simulink model "quadcopter_wind_adaptive_AW"  (R2017b)
settings: Solver=ode45  StartTime=0.0  StopTime=100  FixedStep=0.001  RelTol=1e-3  EnableMultiTasking=on
values from neighbouring files (symbols this model uses):
  aw = 1    [control_params.m]
  C = 1    [control_params.m]
  f_phi = 0.01    [control_params.m]
  f_psi = 0.01    [control_params.m]
  f_theta = 0.01    [control_params.m]
  f_x = 0.01    [control_params.m]
  f_y = 0.01    [control_params.m]
  f_z = 0.01    [control_params.m]
  g = 9.8    [control_params.m]
  J_1 = 0.02    [control_params.m]
  J_2 = 0.02    [control_params.m]
  J_3 = 0.01    [control_params.m]
  l = 0.2    [control_params.m]
  lim_phi = 0.1    [control_params.m]
  lim_psi = 0.1    [control_params.m]
  lim_theta = 0.1    [control_params.m]
  lim_x = 0.1    [control_params.m]
  lim_y = 0.1    [control_params.m]
  lim_z = 6    [control_params.m]
  m = 0.5    [control_params.m]
  phi_desired = 1    [control_params.m]
  x_desired = 1    [control_params.m]
  y_desired = 1    [control_params.m]
  z_desired = 1    [control_params.m]
settings Model: Creator=Oleg Borisov  LastModifiedBy=broth
settings DataIOCC: LimitDataPoints=on  SaveFormat=Array  SignalLoggingSaveFormat=ModelDataLogs
settings OptimizationCC: ExpressionDepthLimit=2147483647  LifeSpan=inf
settings DebuggingCC: UnderspecifiedInitializationDetection=Classic  MergeDetectMultiDrivingBlocksExec=none  SolverPrmCheckMsg=warning  FcnCallInpInsideContextMsg=warning  StateNameClashWarn=warning  SFUnexpectedBacktrackingDiag=warning  SFNoUnconditionalDefaultTransitionDiag=warning  SFExecutionAtInitializationDiag=none
settings HardwareCC: ProdBitPerPointer=32  ProdBitPerSizeT=32  ProdBitPerPtrDiffT=32  ProdLargestAtomicFloat=None  ProdIntDivRoundTo=Undefined  ProdEndianess=Unspecified  ProdWordSize=32  ProdHWDeviceType=32-bit Generic
settings ModelReferenceCC: PropagateSignalLabelsOutOfModel=off
settings CodeAppCC: StateflowObjectComments=on
settings GRTTargetCC: TargetLangStandard=C89/C90 (ANSI)  GeneratePreprocessorConditionals=Disable all  CombineOutputUpdateFcns=off  GRTInterface=on
settings ConfigComp: CovMetricSettings=dw  CovHtmlReporting=on  CovSaveCumulativeToWorkspaceVar=on  CovSaveSingleToWorkspaceVar=on  CovExternalEMLEnable=off  CovSFcnEnable=off

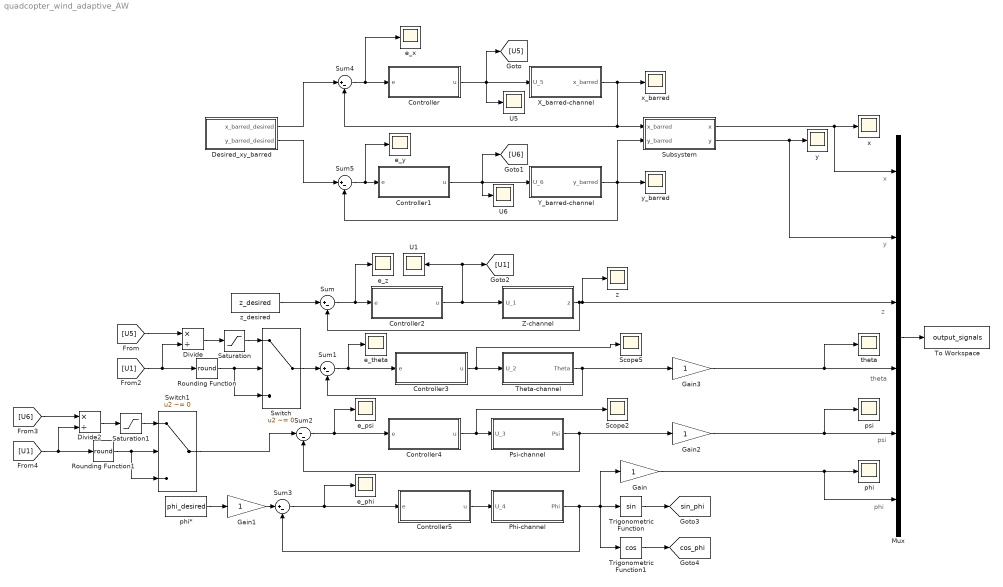
== system quadcopter_wind_adaptive_AW ==
  note: z
  note: y
  note: x
  note: theta
  note: psi
  note: phi
  Controller : Subsystem
  Controller1 : Subsystem
  Controller2 : Subsystem
  Controller3 : Subsystem
  Controller4 : Subsystem
  Controller5 : Subsystem
  Desired_xy_barred : Subsystem
  Divide : Product  Inputs=*/
  Divide2 : Product  Inputs=*/
  Gain{,1..3} (4 alike) : Gain
  Mux : Mux  Inputs=6
  Phi-channel : Subsystem
  Psi-channel : Subsystem
  Rounding Function : Rounding  Operator=round
  Rounding Function1 : Rounding  Operator=round
  Saturation : Saturate  UpperLimit=pi/6  LowerLimit=-pi/6
  Saturation1 : Saturate  UpperLimit=pi/6  LowerLimit=-pi/6
  Scope2 : Scope
  Scope5 : Scope
  Subsystem : Subsystem
  Sum{,1,3..5} (5 alike) : Sum  Inputs=|+-
  Sum2 : Sum  Inputs=|--
  Switch : Switch  Criteria=u2 ~= 0
  Switch1 : Switch  Criteria=u2 ~= 0
  Theta-channel : Subsystem
  To Workspace : ToWorkspace  VariableName=output_signals  SaveFormat=Structure With Time  SampleTime=-1
  Trigonometric Function : Trigonometry
  Trigonometric Function1 : Trigonometry  Operator=cos
  U1 : Scope
  U5 : Scope
  U6 : Scope
  X_barred-channel : Subsystem
  Y_barred-channel : Subsystem
  Z-channel : Subsystem
  e_phi : Scope
  e_psi : Scope
  e_theta : Scope
  e_x : Scope
  e_y : Scope
  e_z : Scope
  phi : Scope
  phi* : Constant  Value=phi_desired
  psi : Scope
  theta : Scope
  x : Scope
  x_barred : Scope
  y : Scope
  y_barred : Scope
  z : Scope
  z_desired : Constant  Value=z_desired
  tag scope: cos_phi=global, sin_phi=global
  wires:
  Z-channel/1(z) -> Mux/3, z/1, Sum/2
  Sum/1 -> Controller2/1(e), e_z/1
  Controller4/1(u) -> Psi-channel/1(U_3), Scope2/1
  Controller5/1(u) -> Phi-channel/1(U_4)
  Theta-channel/1(Theta) -> Sum1/2, Gain3/1
  Sum1/1 -> Controller3/1(e), e_theta/1
  Sum2/1 -> Controller4/1(e), e_psi/1
  Psi-channel/1(Psi) -> Sum2/2, Gain2/1
  Sum3/1 -> Controller5/1(e), e_phi/1
  Phi-channel/1(Phi) -> Sum3/2, Trigonometric Function/1, Trigonometric Function1/1, Gain/1
  Controller1/1(u) -> Y_barred-channel/1(U_6), [U6], U6/1
  [U5] -> Divide/1
  X_barred-channel/1(x_barred) -> x_barred/1, Subsystem/1(x_barred), Sum4/2
  Sum5/1 -> Controller1/1(e), e_y/1
  Y_barred-channel/1(y_barred) -> y_barred/1, Sum5/2, Subsystem/2(y_barred)
  Desired_xy_barred/1(x_barred_desired) -> Sum4/1
  Desired_xy_barred/2(y_barred_desired) -> Sum5/1
  Trigonometric Function/1 -> [sin_phi]
  Trigonometric Function1/1 -> [cos_phi]
  Gain/1 -> Mux/6, phi/1
  phi*/1 -> Gain1/1
  Gain1/1 -> Sum3/1
  Mux/1 -> To Workspace/1
  Subsystem/1(x) -> Mux/1, x/1
  Subsystem/2(y) -> Mux/2, y/1
  Gain2/1 -> Mux/5, psi/1
  Gain3/1 -> Mux/4, theta/1
  Sum4/1 -> Controller/1(e), e_x/1
  Controller/1(u) -> X_barred-channel/1(U_5), [U5], U5/1
  Controller2/1(u) -> Z-channel/1(U_1), [U1], U1/1
  z_desired/1 -> Sum/1
  Divide/1 -> Saturation/1
  [U1] -> Divide/2, Rounding Function/1
  Switch/1 -> Sum1/1
  Saturation/1 -> Switch/1
  Rounding Function/1 -> Switch/2, Switch/3
  Controller3/1(u) -> Theta-channel/1(U_2), Scope5/1
  [U6] -> Divide2/1
  Divide2/1 -> Saturation1/1
  [U1] -> Divide2/2, Rounding Function1/1
  Saturation1/1 -> Switch1/1
  Rounding Function1/1 -> Switch1/2, Switch1/3
  Switch1/1 -> Sum2/1

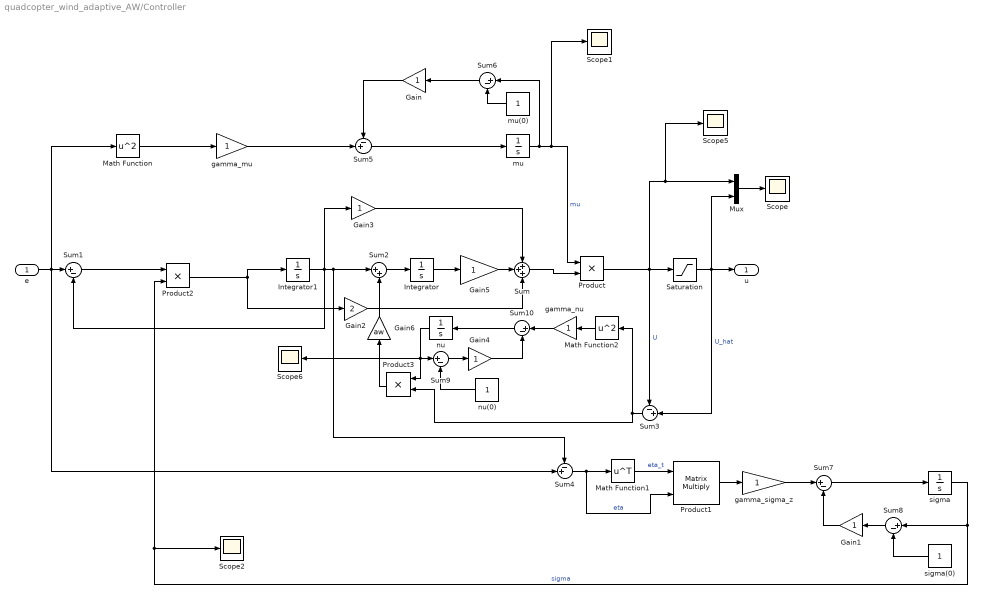
== system quadcopter_wind_adaptive_AW/Controller ==
  e : Inport
  Gain{,1,3..5} (5 alike) : Gain
  Gain2 : Gain  Gain=2
  Gain6 : Gain  Gain=aw
  Integrator : Integrator
  Integrator1 : Integrator
  Math Function : Math  Operator=square  SaturateOnIntegerOverflow=on
  Math Function1 : Math  Operator=transpose  SaturateOnIntegerOverflow=on
  Math Function2 : Math  Operator=square  SaturateOnIntegerOverflow=on
  Mux : Mux  Inputs=2
  Product : Product
  Product1 : Product  Multiplication=Matrix(*)
  Product2 : Product
  Product3 : Product
  Saturation : Saturate  UpperLimit=lim_x  LowerLimit=-lim_x
  Scope{,1..2,5..6} (5 alike) : Scope
  Sum : Sum  Inputs=+++
  Sum{1,6..10} (6 alike) : Sum  Inputs=|+-
  Sum2 : Sum  Inputs=|++
  Sum3 : Sum  Inputs=-+|
  Sum4 : Sum  Inputs=-+|
  Sum5 : Sum  Inputs=-+|
  gamma_mu : Gain
  gamma_nu : Gain
  gamma_sigma_z : Gain
  mu : Integrator  InitialCondition=1
  mu(0) : Constant
  nu : Integrator  InitialCondition=1
  nu(0) : Constant
  sigma : Integrator  InitialCondition=1
  sigma(0) : Constant
  u : Outport
  wires:
  Sum/1 -> Product/2
  Integrator/1 -> Gain5/1
  Sum1/1 -> Product2/1
  Integrator1/1 -> Gain3/1, Sum1/2, Sum4/1, Sum2/1
  Gain3/1 -> Sum/1
  e/1 -> Sum4/2, Math Function/1, Sum1/1
  Gain2/1 -> Sum/3
  Saturation/1 -> u/1, Sum3/2, Mux/2  "U_hat"
  Product/1 -> Saturation/1, Sum3/1, Scope5/1, Mux/1  "U"
  Sum3/1 -> Product3/2, Math Function2/1
  Sum2/1 -> Integrator/1
  Mux/1 -> Scope/1
  Gain5/1 -> Sum/2
  Math Function/1 -> gamma_mu/1
  mu/1 -> Sum6/1, Scope1/1, Product/1  "mu"
  Sum4/1 -> Product1/2, Math Function1/1  "eta"
  Math Function1/1 -> Product1/1  "eta_t"
  Product1/1 -> gamma_sigma_z/1
  sigma/1 -> Sum8/1, Product2/2, Scope2/1  "sigma"
  Product2/1 -> Integrator1/1, Gain2/1
  Math Function2/1 -> gamma_nu/1
  mu(0)/1 -> Sum6/2
  Sum6/1 -> Gain/1
  Gain/1 -> Sum5/1
  gamma_mu/1 -> Sum5/2
  Sum5/1 -> mu/1
  Sum7/1 -> sigma/1
  sigma(0)/1 -> Sum8/2
  Sum8/1 -> Gain1/1
  gamma_sigma_z/1 -> Sum7/1
  Gain1/1 -> Sum7/2
  gamma_nu/1 -> Sum10/1
  Sum10/1 -> nu/1
  nu(0)/1 -> Sum9/2
  Sum9/1 -> Gain4/1
  Gain4/1 -> Sum10/2
  nu/1 -> Scope6/1, Product3/1, Sum9/1
  Product3/1 -> Gain6/1
  Gain6/1 -> Sum2/2

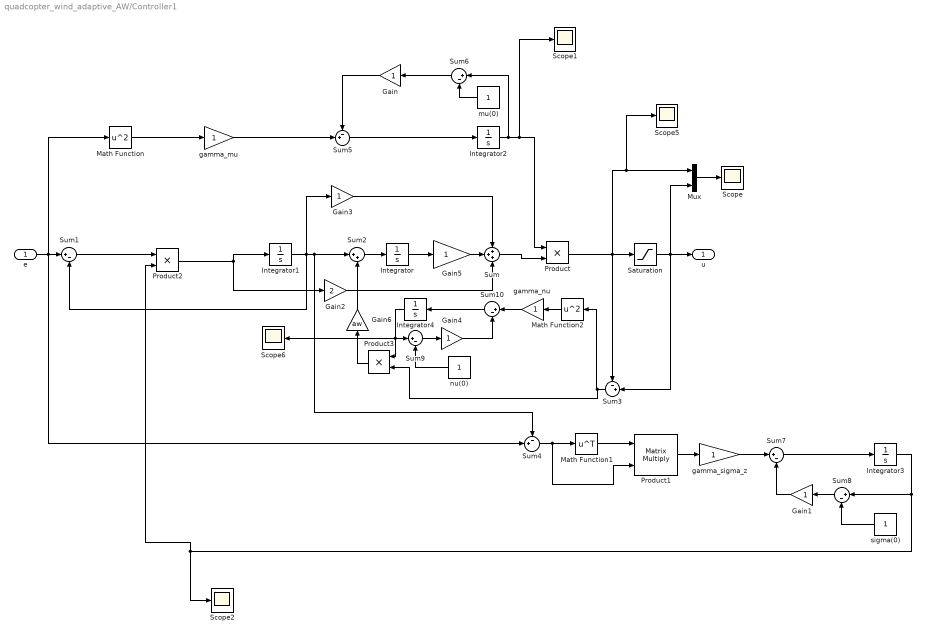
== system quadcopter_wind_adaptive_AW/Controller1 ==
  e : Inport
  Gain{,1,3..5} (5 alike) : Gain
  Gain2 : Gain  Gain=2
  Gain6 : Gain  Gain=aw
  Integrator : Integrator
  Integrator1 : Integrator
  Integrator2 : Integrator  InitialCondition=1
  Integrator3 : Integrator  InitialCondition=1
  Integrator4 : Integrator  InitialCondition=1
  Math Function : Math  Operator=square  SaturateOnIntegerOverflow=on
  Math Function1 : Math  Operator=transpose  SaturateOnIntegerOverflow=on
  Math Function2 : Math  Operator=square  SaturateOnIntegerOverflow=on
  Mux : Mux  Inputs=2
  Product : Product
  Product1 : Product  Multiplication=Matrix(*)
  Product2 : Product
  Product3 : Product
  Saturation : Saturate  UpperLimit=lim_y  LowerLimit=-lim_y
  Scope{,1..2,5..6} (5 alike) : Scope
  Sum : Sum  Inputs=+++
  Sum{1,6..10} (6 alike) : Sum  Inputs=|+-
  Sum2 : Sum  Inputs=|++
  Sum3 : Sum  Inputs=-+|
  Sum4 : Sum  Inputs=-+|
  Sum5 : Sum  Inputs=-+|
  gamma_mu : Gain
  gamma_nu : Gain
  gamma_sigma_z : Gain
  mu(0) : Constant
  nu(0) : Constant
  sigma(0) : Constant
  u : Outport
  wires:
  Sum/1 -> Product/2
  Integrator/1 -> Gain5/1
  Sum1/1 -> Product2/1
  Integrator1/1 -> Gain3/1, Sum1/2, Sum4/1, Sum2/1
  Gain3/1 -> Sum/1
  e/1 -> Sum4/2, Math Function/1, Sum1/1
  Gain2/1 -> Sum/3
  Saturation/1 -> u/1, Sum3/2, Mux/2
  Product/1 -> Saturation/1, Sum3/1, Scope5/1, Mux/1
  Sum3/1 -> Product3/2, Math Function2/1
  Sum2/1 -> Integrator/1
  Mux/1 -> Scope/1
  Gain5/1 -> Sum/2
  Math Function/1 -> gamma_mu/1
  Integrator2/1 -> Sum6/1, Scope1/1, Product/1
  Sum4/1 -> Product1/2, Math Function1/1
  Math Function1/1 -> Product1/1
  Product1/1 -> gamma_sigma_z/1
  Integrator3/1 -> Sum8/1, Product2/2, Scope2/1
  Product2/1 -> Integrator1/1, Gain2/1
  Math Function2/1 -> gamma_nu/1
  mu(0)/1 -> Sum6/2
  Sum6/1 -> Gain/1
  Gain/1 -> Sum5/1
  gamma_mu/1 -> Sum5/2
  Sum5/1 -> Integrator2/1
  Sum7/1 -> Integrator3/1
  sigma(0)/1 -> Sum8/2
  Sum8/1 -> Gain1/1
  gamma_sigma_z/1 -> Sum7/1
  Gain1/1 -> Sum7/2
  gamma_nu/1 -> Sum10/1
  Sum10/1 -> Integrator4/1
  nu(0)/1 -> Sum9/2
  Sum9/1 -> Gain4/1
  Gain4/1 -> Sum10/2
  Integrator4/1 -> Scope6/1, Product3/1, Sum9/1
  Product3/1 -> Gain6/1
  Gain6/1 -> Sum2/2

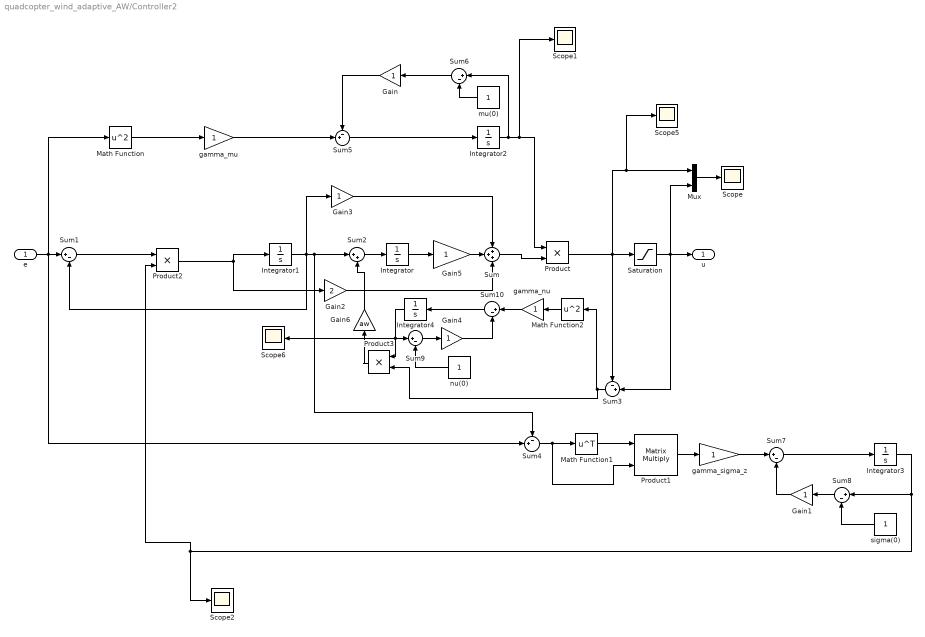
== system quadcopter_wind_adaptive_AW/Controller2 ==
  e : Inport
  Gain{,1,3..5} (5 alike) : Gain
  Gain2 : Gain  Gain=2
  Gain6 : Gain  Gain=aw
  Integrator : Integrator
  Integrator1 : Integrator
  Integrator2 : Integrator  InitialCondition=1
  Integrator3 : Integrator  InitialCondition=1
  Integrator4 : Integrator  InitialCondition=1
  Math Function : Math  Operator=square  SaturateOnIntegerOverflow=on
  Math Function1 : Math  Operator=transpose  SaturateOnIntegerOverflow=on
  Math Function2 : Math  Operator=square  SaturateOnIntegerOverflow=on
  Mux : Mux  Inputs=2
  Product : Product
  Product1 : Product  Multiplication=Matrix(*)
  Product2 : Product
  Product3 : Product
  Saturation : Saturate  UpperLimit=lim_z  LowerLimit=-lim_z
  Scope{,1..2,5..6} (5 alike) : Scope
  Sum : Sum  Inputs=+++
  Sum{1,6..10} (6 alike) : Sum  Inputs=|+-
  Sum2 : Sum  Inputs=|++
  Sum3 : Sum  Inputs=-+|
  Sum4 : Sum  Inputs=-+|
  Sum5 : Sum  Inputs=-+|
  gamma_mu : Gain
  gamma_nu : Gain
  gamma_sigma_z : Gain
  mu(0) : Constant
  nu(0) : Constant
  sigma(0) : Constant
  u : Outport
  wires:
  Sum/1 -> Product/2
  Integrator/1 -> Gain5/1
  Sum1/1 -> Product2/1
  Integrator1/1 -> Gain3/1, Sum1/2, Sum4/1, Sum2/1
  Gain3/1 -> Sum/1
  e/1 -> Sum4/2, Math Function/1, Sum1/1
  Gain2/1 -> Sum/3
  Saturation/1 -> u/1, Sum3/2, Mux/2
  Product/1 -> Saturation/1, Sum3/1, Scope5/1, Mux/1
  Sum3/1 -> Product3/2, Math Function2/1
  Sum2/1 -> Integrator/1
  Mux/1 -> Scope/1
  Gain5/1 -> Sum/2
  Math Function/1 -> gamma_mu/1
  Integrator2/1 -> Sum6/1, Scope1/1, Product/1
  Sum4/1 -> Product1/2, Math Function1/1
  Math Function1/1 -> Product1/1
  Product1/1 -> gamma_sigma_z/1
  Integrator3/1 -> Sum8/1, Product2/2, Scope2/1
  Product2/1 -> Integrator1/1, Gain2/1
  Math Function2/1 -> gamma_nu/1
  mu(0)/1 -> Sum6/2
  Sum6/1 -> Gain/1
  Gain/1 -> Sum5/1
  gamma_mu/1 -> Sum5/2
  Sum5/1 -> Integrator2/1
  Sum7/1 -> Integrator3/1
  sigma(0)/1 -> Sum8/2
  Sum8/1 -> Gain1/1
  gamma_sigma_z/1 -> Sum7/1
  Gain1/1 -> Sum7/2
  gamma_nu/1 -> Sum10/1
  Sum10/1 -> Integrator4/1
  nu(0)/1 -> Sum9/2
  Sum9/1 -> Gain4/1
  Gain4/1 -> Sum10/2
  Integrator4/1 -> Scope6/1, Product3/1, Sum9/1
  Product3/1 -> Gain6/1
  Gain6/1 -> Sum2/2

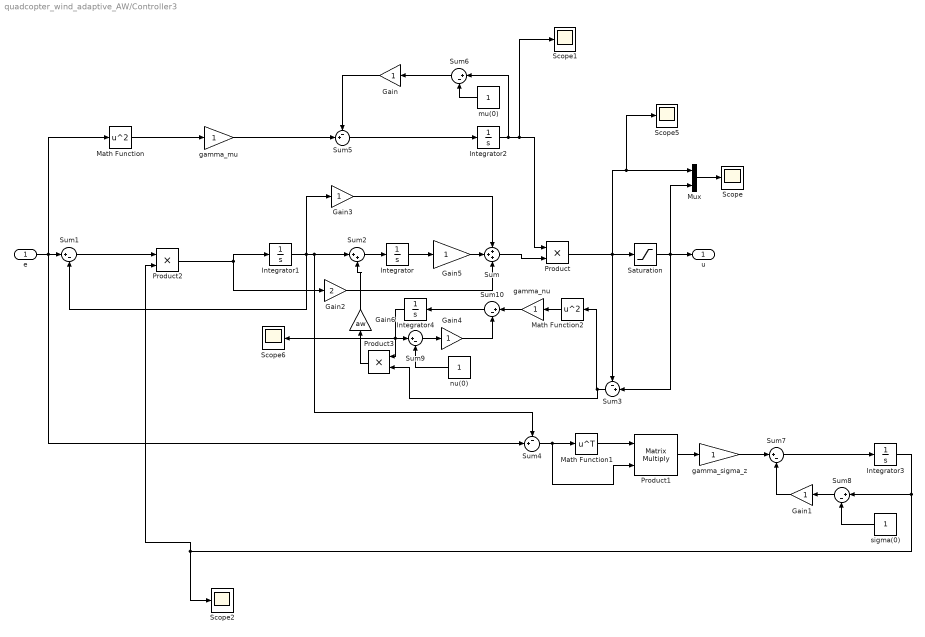
== system quadcopter_wind_adaptive_AW/Controller3 ==
  e : Inport
  Gain{,1,3..5} (5 alike) : Gain
  Gain2 : Gain  Gain=2
  Gain6 : Gain  Gain=aw
  Integrator : Integrator
  Integrator1 : Integrator
  Integrator2 : Integrator  InitialCondition=1
  Integrator3 : Integrator  InitialCondition=1
  Integrator4 : Integrator  InitialCondition=1
  Math Function : Math  Operator=square  SaturateOnIntegerOverflow=on
  Math Function1 : Math  Operator=transpose  SaturateOnIntegerOverflow=on
  Math Function2 : Math  Operator=square  SaturateOnIntegerOverflow=on
  Mux : Mux  Inputs=2
  Product : Product
  Product1 : Product  Multiplication=Matrix(*)
  Product2 : Product
  Product3 : Product
  Saturation : Saturate  UpperLimit=lim_theta  LowerLimit=-lim_theta
  Scope{,1..2,5..6} (5 alike) : Scope
  Sum : Sum  Inputs=+++
  Sum{1,6..10} (6 alike) : Sum  Inputs=|+-
  Sum2 : Sum  Inputs=|++
  Sum3 : Sum  Inputs=-+|
  Sum4 : Sum  Inputs=-+|
  Sum5 : Sum  Inputs=-+|
  gamma_mu : Gain
  gamma_nu : Gain
  gamma_sigma_z : Gain
  mu(0) : Constant
  nu(0) : Constant
  sigma(0) : Constant
  u : Outport
  wires:
  Sum/1 -> Product/2
  Integrator/1 -> Gain5/1
  Sum1/1 -> Product2/1
  Integrator1/1 -> Gain3/1, Sum1/2, Sum4/1, Sum2/1
  Gain3/1 -> Sum/1
  e/1 -> Sum4/2, Math Function/1, Sum1/1
  Gain2/1 -> Sum/3
  Saturation/1 -> u/1, Sum3/2, Mux/2
  Product/1 -> Saturation/1, Sum3/1, Scope5/1, Mux/1
  Sum3/1 -> Product3/2, Math Function2/1
  Sum2/1 -> Integrator/1
  Mux/1 -> Scope/1
  Gain5/1 -> Sum/2
  Math Function/1 -> gamma_mu/1
  Integrator2/1 -> Sum6/1, Scope1/1, Product/1
  Sum4/1 -> Product1/2, Math Function1/1
  Math Function1/1 -> Product1/1
  Product1/1 -> gamma_sigma_z/1
  Integrator3/1 -> Sum8/1, Product2/2, Scope2/1
  Product2/1 -> Integrator1/1, Gain2/1
  Math Function2/1 -> gamma_nu/1
  mu(0)/1 -> Sum6/2
  Sum6/1 -> Gain/1
  Gain/1 -> Sum5/1
  gamma_mu/1 -> Sum5/2
  Sum5/1 -> Integrator2/1
  Sum7/1 -> Integrator3/1
  sigma(0)/1 -> Sum8/2
  Sum8/1 -> Gain1/1
  gamma_sigma_z/1 -> Sum7/1
  Gain1/1 -> Sum7/2
  gamma_nu/1 -> Sum10/1
  Sum10/1 -> Integrator4/1
  nu(0)/1 -> Sum9/2
  Sum9/1 -> Gain4/1
  Gain4/1 -> Sum10/2
  Integrator4/1 -> Scope6/1, Product3/1, Sum9/1
  Product3/1 -> Gain6/1
  Gain6/1 -> Sum2/2

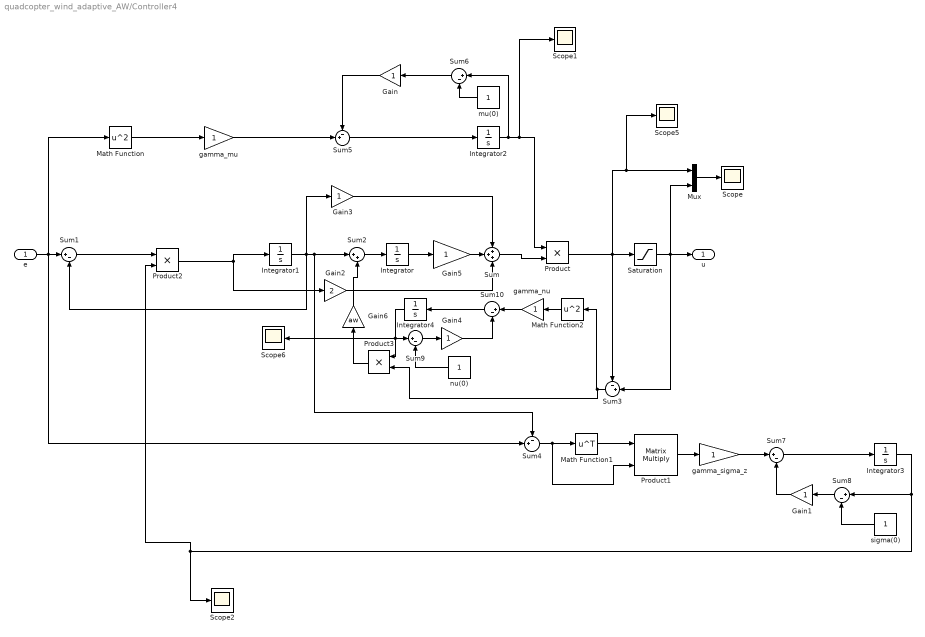
== system quadcopter_wind_adaptive_AW/Controller4 ==
  e : Inport
  Gain{,1,3..5} (5 alike) : Gain
  Gain2 : Gain  Gain=2
  Gain6 : Gain  Gain=aw
  Integrator : Integrator
  Integrator1 : Integrator
  Integrator2 : Integrator  InitialCondition=1
  Integrator3 : Integrator  InitialCondition=1
  Integrator4 : Integrator  InitialCondition=1
  Math Function : Math  Operator=square  SaturateOnIntegerOverflow=on
  Math Function1 : Math  Operator=transpose  SaturateOnIntegerOverflow=on
  Math Function2 : Math  Operator=square  SaturateOnIntegerOverflow=on
  Mux : Mux  Inputs=2
  Product : Product
  Product1 : Product  Multiplication=Matrix(*)
  Product2 : Product
  Product3 : Product
  Saturation : Saturate  UpperLimit=lim_psi  LowerLimit=-lim_psi
  Scope{,1..2,5..6} (5 alike) : Scope
  Sum : Sum  Inputs=+++
  Sum{1,6..10} (6 alike) : Sum  Inputs=|+-
  Sum2 : Sum  Inputs=|++
  Sum3 : Sum  Inputs=-+|
  Sum4 : Sum  Inputs=-+|
  Sum5 : Sum  Inputs=-+|
  gamma_mu : Gain
  gamma_nu : Gain
  gamma_sigma_z : Gain
  mu(0) : Constant
  nu(0) : Constant
  sigma(0) : Constant
  u : Outport
  wires:
  Sum/1 -> Product/2
  Integrator/1 -> Gain5/1
  Sum1/1 -> Product2/1
  Integrator1/1 -> Gain3/1, Sum1/2, Sum4/1, Sum2/1
  Gain3/1 -> Sum/1
  e/1 -> Sum4/2, Math Function/1, Sum1/1
  Gain2/1 -> Sum/3
  Saturation/1 -> u/1, Sum3/2, Mux/2
  Product/1 -> Saturation/1, Sum3/1, Scope5/1, Mux/1
  Sum3/1 -> Product3/2, Math Function2/1
  Sum2/1 -> Integrator/1
  Mux/1 -> Scope/1
  Gain5/1 -> Sum/2
  Math Function/1 -> gamma_mu/1
  Integrator2/1 -> Sum6/1, Scope1/1, Product/1
  Sum4/1 -> Product1/2, Math Function1/1
  Math Function1/1 -> Product1/1
  Product1/1 -> gamma_sigma_z/1
  Integrator3/1 -> Sum8/1, Product2/2, Scope2/1
  Product2/1 -> Integrator1/1, Gain2/1
  Math Function2/1 -> gamma_nu/1
  mu(0)/1 -> Sum6/2
  Sum6/1 -> Gain/1
  Gain/1 -> Sum5/1
  gamma_mu/1 -> Sum5/2
  Sum5/1 -> Integrator2/1
  Sum7/1 -> Integrator3/1
  sigma(0)/1 -> Sum8/2
  Sum8/1 -> Gain1/1
  gamma_sigma_z/1 -> Sum7/1
  Gain1/1 -> Sum7/2
  gamma_nu/1 -> Sum10/1
  Sum10/1 -> Integrator4/1
  nu(0)/1 -> Sum9/2
  Sum9/1 -> Gain4/1
  Gain4/1 -> Sum10/2
  Integrator4/1 -> Scope6/1, Product3/1, Sum9/1
  Product3/1 -> Gain6/1
  Gain6/1 -> Sum2/2

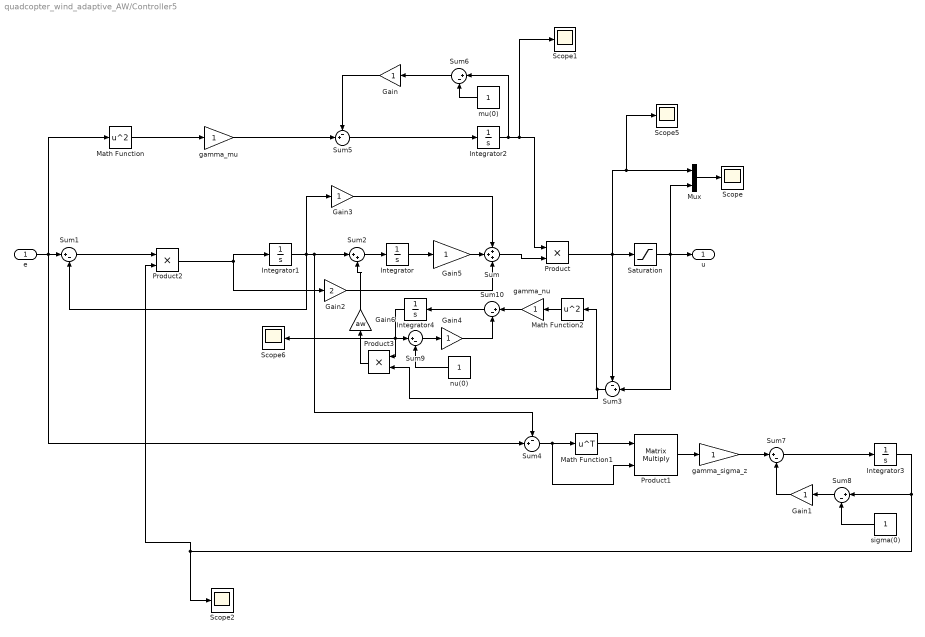
== system quadcopter_wind_adaptive_AW/Controller5 ==
  e : Inport
  Gain{,1,3..5} (5 alike) : Gain
  Gain2 : Gain  Gain=2
  Gain6 : Gain  Gain=aw
  Integrator : Integrator
  Integrator1 : Integrator
  Integrator2 : Integrator  InitialCondition=1
  Integrator3 : Integrator  InitialCondition=1
  Integrator4 : Integrator  InitialCondition=1
  Math Function : Math  Operator=square  SaturateOnIntegerOverflow=on
  Math Function1 : Math  Operator=transpose  SaturateOnIntegerOverflow=on
  Math Function2 : Math  Operator=square  SaturateOnIntegerOverflow=on
  Mux : Mux  Inputs=2
  Product : Product
  Product1 : Product  Multiplication=Matrix(*)
  Product2 : Product
  Product3 : Product
  Saturation : Saturate  UpperLimit=lim_phi  LowerLimit=-lim_phi
  Scope{,1..2,5..6} (5 alike) : Scope
  Sum : Sum  Inputs=+++
  Sum{1,6..10} (6 alike) : Sum  Inputs=|+-
  Sum2 : Sum  Inputs=|++
  Sum3 : Sum  Inputs=-+|
  Sum4 : Sum  Inputs=-+|
  Sum5 : Sum  Inputs=-+|
  gamma_mu : Gain
  gamma_nu : Gain
  gamma_sigma_z : Gain
  mu(0) : Constant
  nu(0) : Constant
  sigma(0) : Constant
  u : Outport
  wires:
  Sum/1 -> Product/2
  Integrator/1 -> Gain5/1
  Sum1/1 -> Product2/1
  Integrator1/1 -> Gain3/1, Sum1/2, Sum4/1, Sum2/1
  Gain3/1 -> Sum/1
  e/1 -> Sum4/2, Math Function/1, Sum1/1
  Gain2/1 -> Sum/3
  Saturation/1 -> u/1, Sum3/2, Mux/2
  Product/1 -> Saturation/1, Sum3/1, Scope5/1, Mux/1
  Sum3/1 -> Product3/2, Math Function2/1
  Sum2/1 -> Integrator/1
  Mux/1 -> Scope/1
  Gain5/1 -> Sum/2
  Math Function/1 -> gamma_mu/1
  Integrator2/1 -> Sum6/1, Scope1/1, Product/1
  Sum4/1 -> Product1/2, Math Function1/1
  Math Function1/1 -> Product1/1
  Product1/1 -> gamma_sigma_z/1
  Integrator3/1 -> Sum8/1, Product2/2, Scope2/1
  Product2/1 -> Integrator1/1, Gain2/1
  Math Function2/1 -> gamma_nu/1
  mu(0)/1 -> Sum6/2
  Sum6/1 -> Gain/1
  Gain/1 -> Sum5/1
  gamma_mu/1 -> Sum5/2
  Sum5/1 -> Integrator2/1
  Sum7/1 -> Integrator3/1
  sigma(0)/1 -> Sum8/2
  Sum8/1 -> Gain1/1
  gamma_sigma_z/1 -> Sum7/1
  Gain1/1 -> Sum7/2
  gamma_nu/1 -> Sum10/1
  Sum10/1 -> Integrator4/1
  nu(0)/1 -> Sum9/2
  Sum9/1 -> Gain4/1
  Gain4/1 -> Sum10/2
  Integrator4/1 -> Scope6/1, Product3/1, Sum9/1
  Product3/1 -> Gain6/1
  Gain6/1 -> Sum2/2

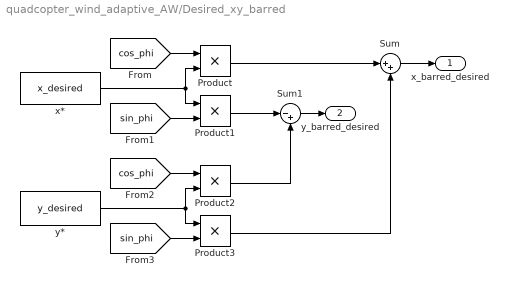
== system quadcopter_wind_adaptive_AW/Desired_xy_barred ==
  Product{,1..3} (4 alike) : Product  RndMeth=Zero
  Sum : Sum  Inputs=|++
  Sum1 : Sum  Inputs=|-+
  x* : Constant  Value=x_desired
  y* : Constant  Value=y_desired
  x_barred_desired : Outport
  y_barred_desired : Outport  Port=2
  wires:
  [cos_phi] -> Product/1
  [sin_phi] -> Product1/2
  [cos_phi] -> Product2/1
  [sin_phi] -> Product3/2
  Product/1 -> Sum/1
  Product3/1 -> Sum/2
  Product1/1 -> Sum1/1
  Product2/1 -> Sum1/2
  Sum/1 -> x_barred_desired/1
  Sum1/1 -> y_barred_desired/1
  x*/1 -> Product/2, Product1/1
  y*/1 -> Product2/2, Product3/1

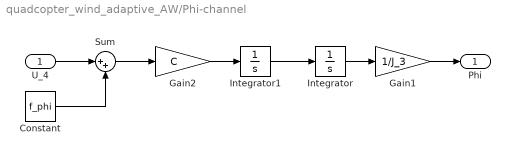
== system quadcopter_wind_adaptive_AW/Phi-channel ==
  U_4 : Inport
  Constant : Constant  Value=f_phi
  Gain1 : Gain  Gain=1/J_3
  Gain2 : Gain  Gain=C
  Integrator : Integrator
  Integrator1 : Integrator
  Sum : Sum  Inputs=|++
  Phi : Outport
  wires:
  Integrator1/1 -> Integrator/1
  Integrator/1 -> Gain1/1
  Gain1/1 -> Phi/1
  Gain2/1 -> Integrator1/1
  U_4/1 -> Sum/1
  Sum/1 -> Gain2/1
  Constant/1 -> Sum/2

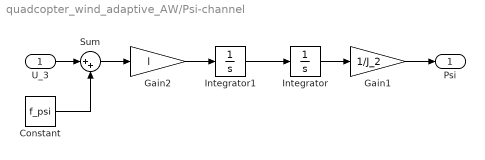
== system quadcopter_wind_adaptive_AW/Psi-channel ==
  U_3 : Inport
  Constant : Constant  Value=f_psi
  Gain1 : Gain  Gain=1/J_2
  Gain2 : Gain  Gain=l
  Integrator : Integrator
  Integrator1 : Integrator
  Sum : Sum  Inputs=|++
  Psi : Outport
  wires:
  Integrator1/1 -> Integrator/1
  Integrator/1 -> Gain1/1
  Gain1/1 -> Psi/1
  Gain2/1 -> Integrator1/1
  U_3/1 -> Sum/1
  Sum/1 -> Gain2/1
  Constant/1 -> Sum/2

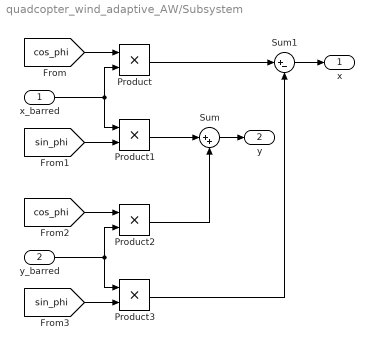
== system quadcopter_wind_adaptive_AW/Subsystem ==
  x_barred : Inport
  y_barred : Inport  Port=2
  Product{,1..3} (4 alike) : Product  RndMeth=Zero
  Sum : Sum  Inputs=|++
  Sum1 : Sum  Inputs=|+-
  x : Outport
  y : Outport  Port=2
  wires:
  [cos_phi] -> Product/1
  [sin_phi] -> Product1/2
  x_barred/1 -> Product/2, Product1/1
  [cos_phi] -> Product2/1
  [sin_phi] -> Product3/2
  y_barred/1 -> Product2/2, Product3/1
  Product1/1 -> Sum/1
  Product2/1 -> Sum/2
  Product/1 -> Sum1/1
  Product3/1 -> Sum1/2
  Sum1/1 -> x/1
  Sum/1 -> y/1

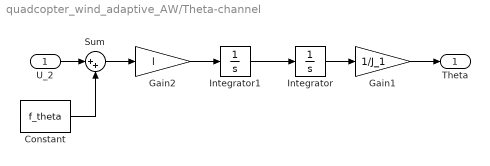
== system quadcopter_wind_adaptive_AW/Theta-channel ==
  U_2 : Inport
  Constant : Constant  Value=f_theta
  Gain1 : Gain  Gain=1/J_1
  Gain2 : Gain  Gain=l
  Integrator : Integrator
  Integrator1 : Integrator
  Sum : Sum  Inputs=|++
  Theta : Outport
  wires:
  Integrator1/1 -> Integrator/1
  Integrator/1 -> Gain1/1
  Gain1/1 -> Theta/1
  Gain2/1 -> Integrator1/1
  U_2/1 -> Sum/1
  Sum/1 -> Gain2/1
  Constant/1 -> Sum/2

== system quadcopter_wind_adaptive_AW/X_barred-channel ==
  U_5 : Inport
  Constant : Constant  Value=f_x
  Gain1 : Gain  Gain=1/m
  Integrator : Integrator
  Integrator1 : Integrator
  Sum : Sum  Inputs=|++
  x_barred : Outport
  wires:
  Integrator1/1 -> Integrator/1
  Integrator/1 -> Gain1/1
  Gain1/1 -> x_barred/1
  U_5/1 -> Sum/1
  Sum/1 -> Integrator1/1
  Constant/1 -> Sum/2

== system quadcopter_wind_adaptive_AW/Y_barred-channel ==
  U_6 : Inport
  Constant : Constant  Value=f_y
  Gain1 : Gain  Gain=1/m
  Integrator : Integrator
  Integrator1 : Integrator
  Sum : Sum  Inputs=|++
  y_barred : Outport
  wires:
  Integrator1/1 -> Integrator/1
  Integrator/1 -> Gain1/1
  Gain1/1 -> y_barred/1
  U_6/1 -> Sum/1
  Sum/1 -> Integrator1/1
  Constant/1 -> Sum/2

== system quadcopter_wind_adaptive_AW/Z-channel ==
  U_1 : Inport
  Constant : Constant  Value=m*g
  Constant1 : Constant  Value=f_z
  Gain1 : Gain  Gain=1/m
  Integrator : Integrator
  Integrator1 : Integrator
  Sum : Sum  Inputs=++-
  z : Outport
  wires:
  Sum/1 -> Integrator1/1
  Integrator1/1 -> Integrator/1
  Integrator/1 -> Gain1/1
  Gain1/1 -> z/1
  Constant/1 -> Sum/3
  U_1/1 -> Sum/2
  Constant1/1 -> Sum/1
